simulink model "exampleRelHum2x"  (Simulink 7.6)
settings: Solver=ode45  StartTime=0.0  StopTime=10.0  RelTol=1e-3
libraries: simulink x3, carnot x1
settings Model: Creator=drhf  LastModifiedBy=drhf

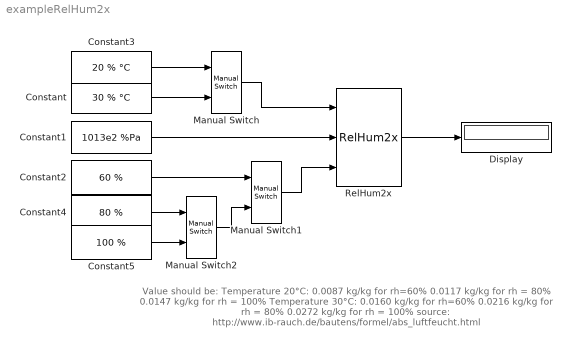
== system exampleRelHum2x ==
  note: Value should be:
      | Temperature 20°C:
      |     0.0087 kg/kg for rh=60%
      |     0.0117 kg/kg for rh = 80%
      |     0.0147 kg/kg for rh = 100%
      | Temperature 30°C:
      |     0.0160 kg/kg for rh=60%
      |     0.0216 kg/kg for rh = 80%
      |     0.0272 kg/kg for rh = 100%
      |
      | source:
      | http://www.ib-rauch.de/bautens/formel/abs_luftfeucht.html
  Constant : Constant  Value=30 % °C
  Constant1 : Constant  Value=1013e2 %Pa
  Constant2 : Constant  Value=60 %
  Constant3 : Constant  Value=20 % °C
  Constant4 : Constant  Value=80 %
  Constant5 : Constant  Value=100 %
  Display : Display
  Manual Switch : simulink/Signal Routing/Manual Switch  SystemSampleTime=-1  sw=0  action=0  varsize=off
  Manual Switch1 : simulink/Signal Routing/Manual Switch  SystemSampleTime=-1  sw=1  action=0  varsize=off
  Manual Switch2 : simulink/Signal Routing/Manual Switch  SystemSampleTime=-1  sw=1  action=0  varsize=off
  RelHum2x : carnot/Basic/Material_Properties/RelHum2x  SystemSampleTime=-1
  wires:
  Constant1/1 -> RelHum2x/2
  RelHum2x/1 -> Display/1
  Constant3/1 -> Manual Switch/1
  Constant/1 -> Manual Switch/2
  Manual Switch/1 -> RelHum2x/1
  Constant4/1 -> Manual Switch2/1
  Constant5/1 -> Manual Switch2/2
  Constant2/1 -> Manual Switch1/1
  Manual Switch2/1 -> Manual Switch1/2
  Manual Switch1/1 -> RelHum2x/3
